simulink model "Q4"  (R2020b)
settings: Solver=VariableStepAuto  StartTime=0.0  StopTime=10.0  RelTol=1e-3
settings Model: Creator=DELL  LastModifiedBy=DELL

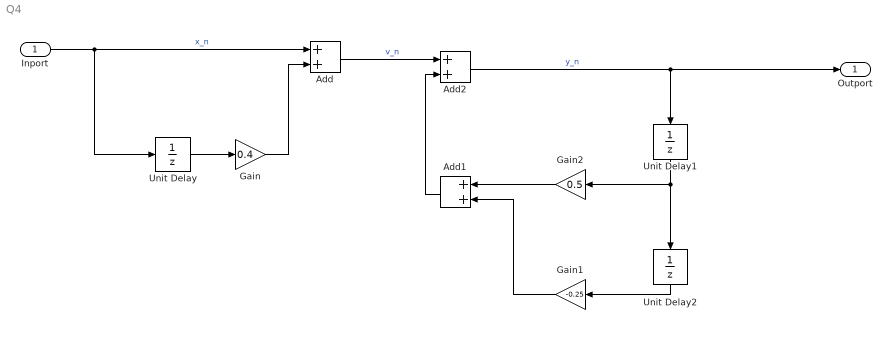
== system Q4 ==
  Inport : Inport
  Add : Sum
  Add1 : Sum
  Add2 : Sum
  Gain : Gain  Gain=0.4
  Gain1 : Gain  Gain=-0.25
  Gain2 : Gain  Gain=0.5
  Unit Delay : UnitDelay  SampleTime=-1  HasFrameUpgradeWarning=on
  Unit Delay1 : UnitDelay  SampleTime=-1  HasFrameUpgradeWarning=on
  Unit Delay2 : UnitDelay  SampleTime=-1  HasFrameUpgradeWarning=on
  Outport : Outport
  wires:
  Gain/1 -> Add/2
  Inport/1 -> Unit Delay/1, Add/1  "x_n"
  Unit Delay/1 -> Gain/1
  Add/1 -> Add2/1  "v_n"
  Gain2/1 -> Add1/1
  Add2/1 -> Unit Delay1/1, Outport/1  "y_n"
  Unit Delay1/1 -> Gain2/1, Unit Delay2/1
  Unit Delay2/1 -> Gain1/1
  Gain1/1 -> Add1/2
  Add1/1 -> Add2/2
